simulink model "IMRFO"  (R2020a)
settings: Solver=VariableStepAuto  StartTime=0.0  StopTime=10  FixedStep=0.001  RelTol=1e-3
values from neighbouring files (symbols this model uses):
  k1 = param1    [BenFunctions.m]
  k2 = param2    [BenFunctions.m]
  k3 = param3    [BenFunctions.m]
undefined symbols (not defined in the file or in its folder): Matlab_version, Output_File, Output_file_n, Plant_inputs_num, Plant_outputs_num, RecurDyn, RecurDyn_controltimestep, RecurDyn_model, RecurDyn_model_n
settings Model: Creator=Karry Wa  LastModifiedBy=lx

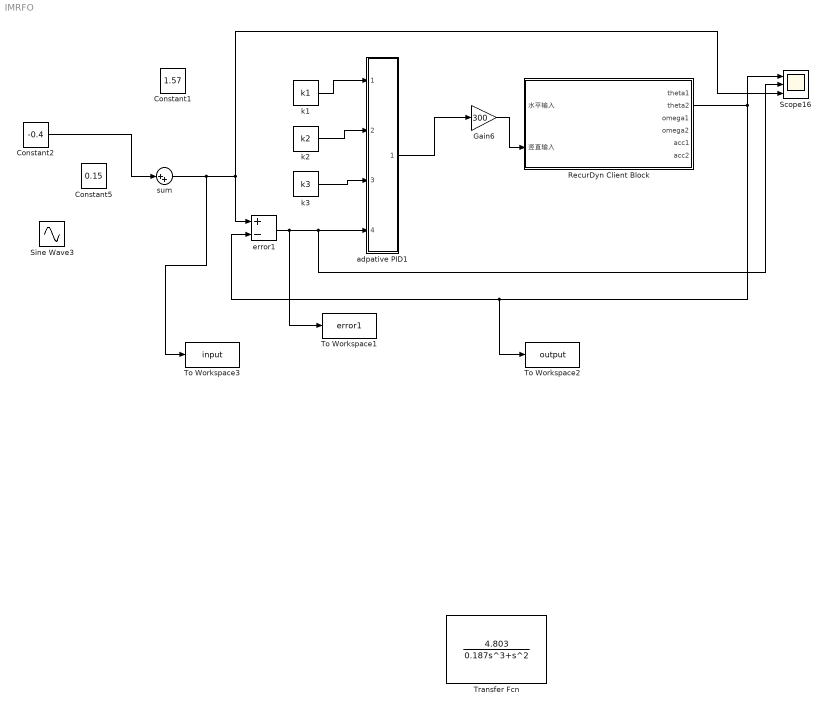
== system IMRFO ==
  Constant1 : Constant  Value=1.57
  Constant2 : Constant  Value=-0.4
  Constant5 : Constant  Value=0.15
  Gain6 : Gain  Gain=300
  RecurDyn Client Block : Subsystem
      mask Display: image(imread('RecurDyn_IF3x_Client.jpg'))
  Scope16 : Scope  NumInputPorts=3
  Sine Wave3 : Sin  Amplitude=0.1  Frequency=6  SampleTime=0
  To Workspace1 : ToWorkspace  VariableName=error1  SampleTime=-1
      settings: Save2DSignal=2-D array (concatenate along first dimension)
  To Workspace2 : ToWorkspace  VariableName=output  SampleTime=-1
      settings: Save2DSignal=2-D array (concatenate along first dimension)
  To Workspace3 : ToWorkspace  VariableName=input  SampleTime=-1
      settings: Save2DSignal=2-D array (concatenate along first dimension)
  Transfer Fcn : TransferFcn  Numerator=4.803  Denominator=[0.187 1 0 0]
  adpative PID1 : Subsystem
  error1 : Sum  Inputs=+-
  k1 : Constant  Value=k1
  k2 : Constant  Value=k2
  k3 : Constant  Value=k3
  sum : Sum  Inputs=|++
  wires:
  adpative PID1/1(Out1) -> Gain6/1
  Gain6/1 -> RecurDyn Client Block/2(竖直输入)
  sum/1 -> To Workspace3/1, Scope16/3, error1/1
  error1/1 -> To Workspace1/1, Scope16/2, adpative PID1/4(In4)
  k1/1 -> adpative PID1/1(In3)
  k2/1 -> adpative PID1/2(In2)
  RecurDyn Client Block/2(theta2) -> To Workspace2/1, error1/2, Scope16/1
  k3/1 -> adpative PID1/3(In1)
  Constant2/1 -> sum/1

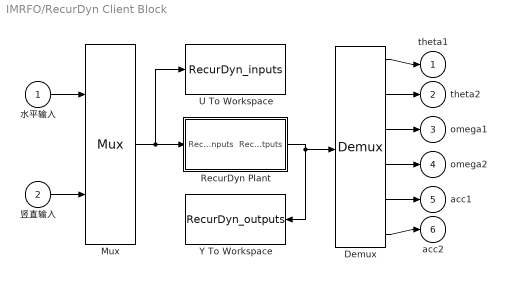
== system IMRFO/RecurDyn Client Block ==
  水平输入 : Inport
  竖直输入 : Inport  Port=2
  Demux : Demux  Outputs=6
      settings: DisplayOption=none
  Mux : Mux  Inputs=2
  RecurDyn Plant : Subsystem  mask(Recurdyn/Plant){RecurDyn_model_name=RecurDyn_model, Output_File_Name_=Output_File, RecurDyn_=RecurDyn, Matlab_version_=Matlab_version, RecurDyn_controltimestep_=RecurDyn_controltimestep, RecurDyn_step_=100, Waitingtime=1000, RecurDyn_static_=off, RecurDyn_show_=on, RecurDyn_ani_=on, Create_Output_Folder_=off}
      mask prompts: Output_File_Name_ "Output File Name"; RecurDyn_ "RecurDyn_install_directory"; Matlab_version_ "Matlab version"; RecurDyn_controltimestep_ "Sampling period"; RecurDyn_step_ "RecurDyn_step"; Waitingtime "Waiting time"; RecurDyn_static_ "Static analysis"; RecurDyn_show_ "RecurDyn_show"; RecurDyn_ani_ "RecurDyn_animation"; Create_Output_Folder_ "Create Output Folder"
      mask help:
      | Simulate any Recurdyn Dynamics Model in Recurdyn/Solver
      | Plant inputs and Plant outputs are transfered every sampling time
      | Here, sampling time is determined by sampling period (Control time step)
      mask Display: disp( 'Dynamic Model' )
  U To Workspace : ToWorkspace  VariableName=RecurDyn_inputs
  Y To Workspace : ToWorkspace  VariableName=RecurDyn_outputs
  theta1 : Outport
  theta2 : Outport  Port=2
  omega1 : Outport  Port=3
  omega2 : Outport  Port=4
  "acc1  " : Outport  Port=5
  "acc2  " : Outport  Port=6
  wires:
  RecurDyn Plant/1(RecurDyn_outputs) -> Demux/1, Y To Workspace/1
  Mux/1 -> RecurDyn Plant/1(" RecurDyn_inputs"), U To Workspace/1
  Demux/1 -> theta1/1
  Demux/2 -> theta2/1
  Demux/3 -> omega1/1
  Demux/4 -> omega2/1
  Demux/5 -> "acc1  "/1
  Demux/6 -> "acc2  "/1
  水平输入/1 -> Mux/1
  竖直输入/1 -> Mux/2

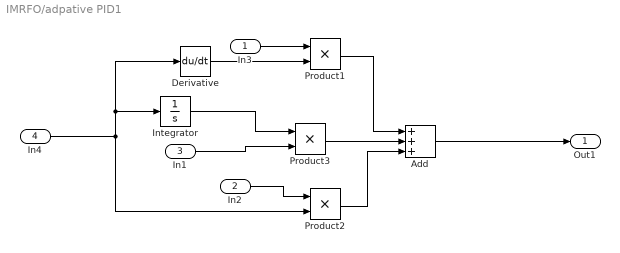
== system IMRFO/adpative PID1 ==
  In3 : Inport
  In2 : Inport  Port=2
  In1 : Inport  Port=3
  In4 : Inport  Port=4
  Add : Sum  Inputs=+++
  Derivative : Derivative
  Integrator : Integrator
  Product1 : Product
  Product2 : Product
  Product3 : Product
  Out1 : Outport
  wires:
  In2/1 -> Product2/1
  In4/1 -> Derivative/1, Integrator/1, Product2/2
  Product1/1 -> Add/1
  Product2/1 -> Add/3
  Derivative/1 -> Product1/2
  In3/1 -> Product1/1
  Add/1 -> Out1/1
  Product3/1 -> Add/2
  In1/1 -> Product3/2
  Integrator/1 -> Product3/1

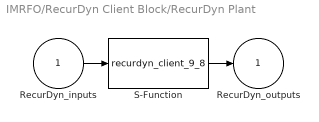
== system IMRFO/RecurDyn Client Block/RecurDyn Plant ==
  " RecurDyn_inputs" : Inport
  S-Function : S-Function  FunctionName=recurdyn_client_9_8  Parameters=RecurDyn_controltimestep_,RecurDyn_model_name,RecurDyn_,RecurDyn_static_,RecurDyn_step_,RecurDyn_show_,RecurDyn_ani_,Matlab_version_,RecurDyn_model_n,Plant_inputs_num,Plant_outputs_num,Waitingtime,Create_Output_Folder_,Output_File_Name_,Output_file_n  SFunctionDeploymentMode=off  EnableBusSupport=off
  RecurDyn_outputs : Outport  InitialOutput=0
  wires:
  S-Function/1 -> RecurDyn_outputs/1
  " RecurDyn_inputs"/1 -> S-Function/1
